simulink model "testHierCtrl"  (R2020a)
settings: Solver=ode23s  StartTime=0.0  StopTime=25  RelTol=1e-3
undefined symbols (not defined in the file or in its folder): a, courseFollowManta, courseFollowManta_cl, env, FLIGHTCONTROLLER, fltCtrl, hiLvlCtrl, initializeBussesFromBlock, vhcl
libraries: simulink x6, angleBtw2Vecs_ul x4, pathGeometry_ul x3, tanFrameProjection_ul x2, vectorNormalizer_ul x2, filteredPIDController_ul x2, velocityAngle_ul x2, eeGeneralControl x1, stopwatch_ul x1, ctrlAllocMatrix_cl x1, eulAng2RotMat_ul x1, vrlib x1
settings Model: Creator=andre  LastModifiedBy=andre
settings DataIOCC: SaveFormat=Structure

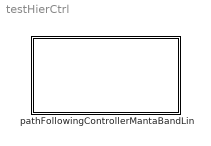
== system testHierCtrl ==
  pathFollowingControllerMantaBandLin : Subsystem  LoadFcn=initializeBussesFromBlock(gcb)  InitFcn=initializeBussesFromBlock(gcb)  StartFcn=initializeBussesFromBlock(gcb)  VariantControl=strcmpi(FLIGHTCONTROLLER,'pathFollowingControllerMantaBandLin')  mask{initPosForInitSStar=vhcl.initPosVecGnd.Value, fluidDensity=env.water.density.Value, pathCtrl=fltCtrl, aeroStruct=vhcl.struct('OCT.aeroSurf')}
      mask prompts: initPosForInitSStar "Initial Position"; fluidDensity "Fluid Density"; pathCtrl "Controller"; aeroStruct "Aerodynamic Structure"
      settings: MinAlgLoopOccurrences=on
      mask DialogControl Container3 Prompt: courseFollow Params
      mask DialogControl Container4 Prompt: setpointToOutput Params

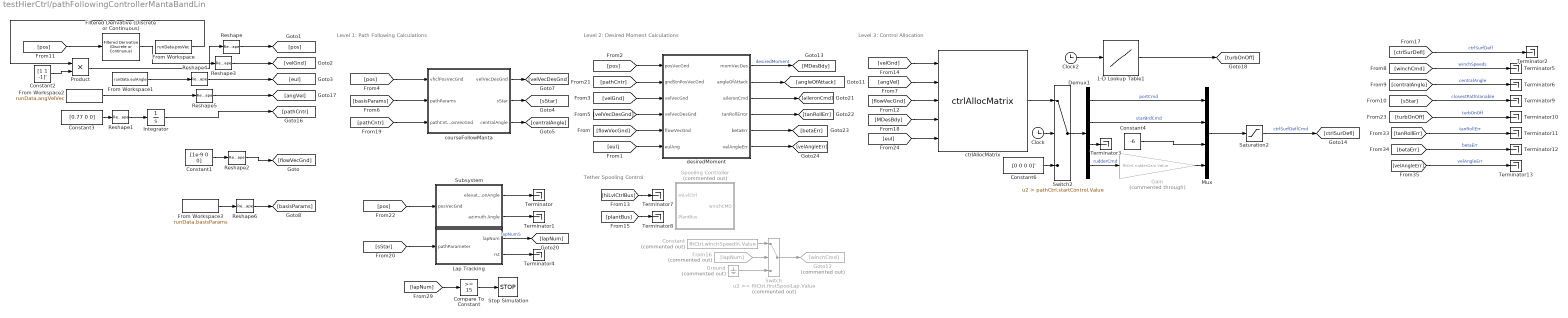
== system testHierCtrl/pathFollowingControllerMantaBandLin ==
  note: Level 1: Path Following Calculations
  note: Level 2: Desired Moment Calculations
  note: Tether Spooling Control
  note: Level 3: Control Allocation
  1-D Lookup Table1 : Lookup_n-D  NumberOfTableDimensions=1  BreakpointsForDimension1=[0 1000 2000]  Table=[0 0 0]  InterpMethod=Flat  InternalRulePriority=Speed  RndMeth=Simplest  InputSameDT=on
  Clock : Clock
  Clock2 : Clock
  Compare To Constant : simulink/Logic and Bit Operations/Compare To Constant  relop=>=  const=15  OutDataTypeStr=boolean
  Constant : Constant  Commented=on  Value=fltCtrl.winchSpeedIn.Value
  Constant1 : Constant  Value=[1e-9 0 0]
  Constant2 : Constant  Value=[1 1 -1]'
  Constant3 : Constant  Value=[0.77 0 0]
  Constant4 : Constant  Value=-6
  Constant6 : Constant  Value=[0 0 0 0]'
  Demux1 : Demux
  Filtered Derivative (Discrete or Continuous) : eeGeneralControl/Filtered Derivative (Discrete or Continuous)  K=1  T=0.1  B=inf  A=-inf  minRatio=10  init_option=Inherited from block input  x0=0  Ts=-1
      settings: SourceProductBaseCode=PS
  From Workspace : FromWorkspace  VariableName=runData.posVec
  From Workspace1 : FromWorkspace  VariableName=runData.eulAngle
  From Workspace2 : FromWorkspace  VariableName=runData.angVelVec
  From Workspace3 : FromWorkspace  VariableName=runData.basisParams
  From16 : From  Commented=on  GotoTag=lapNum
  Gain : Gain  Commented=through  Gain=fltCtrl.rudderGain.Value
  Goto12 : Goto  Commented=on  GotoTag=winchCmd
  Ground : Ground  Commented=on
  Integrator : Integrator  InitialCondition=[0 0 0]'
  Lap Tracking : Subsystem
  Mux : Mux
  Product : Product
  Reshape{,1..6} (7 alike) : Reshape  OutputDimensionality=Column vector (2-D)
  Saturation2 : Saturate  UpperLimit=pathCtrl.controlSigMax.upperLimit.Value  LowerLimit=pathCtrl.controlSigMax.lowerLimit.Value
  "Spooling Controller " : Subsystem  Commented=on
  Stop Simulation : Stop
  Subsystem : Subsystem
  Switch : Switch  Commented=on  Threshold=fltCtrl.firstSpoolLap.Value
  Switch2 : Switch  Criteria=u2 > Threshold  Threshold=pathCtrl.startControl.Value
  Terminator{,1..13} (14 alike) : Terminator
  courseFollowManta : Subsystem  AncestorBlock=courseFollowManta_cl/courseFollowManta
  ctrlAllocMatrix : ctrlAllocMatrix_cl/ctrlAllocMatrix  aeroStruct=aeroStruct  fluidDensity=fluidDensity
  desiredMoment : Subsystem
  wires:
  [velAngleErr] -> Terminator13/1  "velAngleErr"
  desiredMoment/6(velAngleErr) -> [velAngleErr]
  [betaErr] -> Terminator12/1  "betaErr"
  [tanRollErr] -> Terminator11/1  "tanRollErr"
  desiredMoment/5(betaErr) -> [betaErr]
  desiredMoment/4(tanRollError) -> [tanRollErr]
  Mux/1 -> Saturation2/1
  desiredMoment/3(aileronCmd) -> [aileronCmd]
  Compare To Constant/1 -> Stop Simulation/1
  [lapNum] -> Compare To Constant/1
  Ground/1 -> Switch/3
  Constant/1 -> Switch/1
  From16/1 -> Switch/2
  Switch/1 -> Goto12/1
  [plantBus] -> Terminator8/1
  [hiLvlCtrlBus] -> Terminator7/1
  Lap Tracking/1(lapNum) -> [lapNum]  "lapNumS"
  Lap Tracking/2(rst) -> Terminator4/1
  [sStar] -> Lap Tracking/1(pathParameter)
  Clock2/1 -> 1-D Lookup Table1/1
  1-D Lookup Table1/1 -> [turbOnOff]
  desiredMoment/2(angleOfAttack) -> [angleOfAttack]
  Constant4/1 -> Mux/3
  Subsystem/2(azimuth Angle) -> Terminator1/1
  Subsystem/1(elevationAngle) -> Terminator/1
  [pos] -> Subsystem/1(posVecGnd)
  [turbOnOff] -> Terminator10/1  "turbOnOff"
  Demux1/4 -> Gain/1  "rudderCmd"
  Gain/1 -> Mux/4
  [basisParams] -> courseFollowManta/2(pathParams)
  [flowVecGnd] -> desiredMoment/5(flowVecGnd)
  [eul] -> desiredMoment/6(eulAng)
  [velVecDesGnd] -> desiredMoment/4(velVecDesGnd)
  [velGnd] -> desiredMoment/3(velVecGnd)
  [pathCntr] -> desiredMoment/2(gndStnPosVecGnd)
  [pos] -> desiredMoment/1(posVecGnd)
  [pathCntr] -> courseFollowManta/3(pathCntrPosVecGnd)
  [eul] -> ctrlAllocMatrix/5
  Saturation2/1 -> [ctrlSurDefl]  "ctrlSurfDeflCmd"
  [ctrlSurDefl] -> Terminator2/1  "ctrlSurfDefl"
  ctrlAllocMatrix/1 -> Switch2/1
  [MDesBdy] -> ctrlAllocMatrix/4
  Constant6/1 -> Switch2/3
  Switch2/1 -> Demux1/1
  Clock/1 -> Switch2/2
  Demux1/2 -> Mux/2  "starBrdCmd"
  Demux1/1 -> Mux/1  "portCmd"
  Demux1/3 -> Terminator3/1
  [flowVecGnd] -> ctrlAllocMatrix/3
  [velGnd] -> ctrlAllocMatrix/1
  [angVel] -> ctrlAllocMatrix/2
  desiredMoment/1(momVecDes) -> [MDesBdy]  "desiredMoment"
  courseFollowManta/3(centralAngle) -> [centralAngle]
  [sStar] -> Terminator9/1  "closestPathVariable"
  [centralAngle] -> Terminator6/1  "centralAngle"
  courseFollowManta/2(sStar) -> [sStar]
  [winchCmd] -> Terminator5/1  "winchSpeeds"
  [pos] -> courseFollowManta/1("vhclPosVecGnd ")
  courseFollowManta/1(velVecDesGnd) -> [velVecDesGnd]
  From Workspace/1 -> Product/1
  Reshape3/1 -> [velGnd]
  Filtered Derivative (Discrete or Continuous)/1 -> Reshape3/1
  From Workspace1/1 -> Reshape4/1
  Constant3/1 -> Reshape1/1
  Reshape1/1 -> Integrator/1
  Integrator/1 -> [pathCntr]
  Constant1/1 -> Reshape2/1
  Reshape2/1 -> [flowVecGnd]
  Reshape/1 -> [pos]
  [pos] -> Filtered Derivative (Discrete or Continuous)/1
  From Workspace2/1 -> Reshape5/1
  From Workspace3/1 -> Reshape6/1
  Reshape4/1 -> [eul]
  Reshape5/1 -> [angVel]
  Reshape6/1 -> [basisParams]
  Constant2/1 -> Product/2
  Product/1 -> Reshape/1

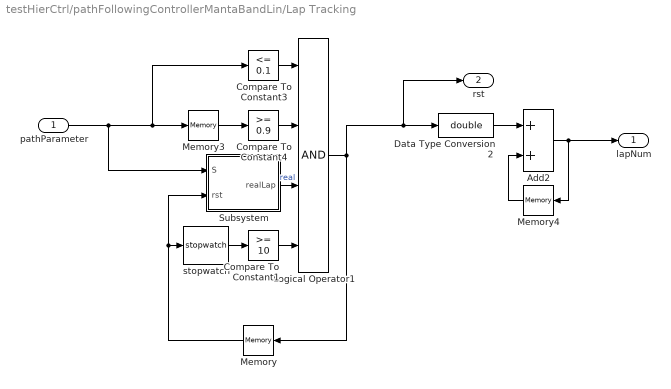
== system testHierCtrl/pathFollowingControllerMantaBandLin/Lap Tracking ==
  pathParameter : Inport
  Add2 : Sum
  Compare To Constant1 : simulink/Logic and Bit Operations/Compare To Constant  relop=>=  const=10  OutDataTypeStr=boolean
  Compare To Constant3 : simulink/Logic and Bit Operations/Compare To Constant  relop=<=  const=0.1  OutDataTypeStr=boolean
  Compare To Constant4 : simulink/Logic and Bit Operations/Compare To Constant  relop=>=  const=0.9  OutDataTypeStr=boolean
  Data Type Conversion2 : DataTypeConversion  OutDataTypeStr=double
  Logical Operator1 : Logic  Inputs=4  AllPortsSameDT=off  OutDataTypeStr=boolean
  Memory : Memory  InitialCondition=false
  Memory3 : Memory
  Memory4 : Memory
  Subsystem : Subsystem
  stopwatch : stopwatch_ul/stopwatch  SystemSampleTime=-1  Latency=0  AutoFrameSizeCalculation=off
  lapNum : Outport  VectorParamsAs1DForOutWhenUnconnected=off
  rst : Outport  Port=2  VectorParamsAs1DForOutWhenUnconnected=off
  wires:
  Subsystem/1(realLap) -> Logical Operator1/3  "real"
  Compare To Constant1/1 -> Logical Operator1/4
  Memory/1 -> stopwatch/1, Subsystem/2(rst)
  stopwatch/1 -> Compare To Constant1/1
  pathParameter/1 -> Memory3/1, Compare To Constant3/1, Subsystem/1(S)
  Compare To Constant4/1 -> Logical Operator1/2
  Add2/1 -> Memory4/1, lapNum/1
  Memory4/1 -> Add2/2
  Logical Operator1/1 -> Memory/1, Data Type Conversion2/1, rst/1
  Data Type Conversion2/1 -> Add2/1
  Memory3/1 -> Compare To Constant4/1
  Compare To Constant3/1 -> Logical Operator1/1

== system testHierCtrl/pathFollowingControllerMantaBandLin/Spooling Controller  ==
  HiLvlCtrl : Inport
  PlantBus : Inport  Port=2
  Add1 : Sum  Inputs=+-
  Bus Selector1 : BusSelector  OutputSignals=avgTetherLength
  Bus Selector3 : BusSelector  OutputSignals=basisParams
  Constant2 : Constant  Value=fltCtrl.optAltitude.Value
  Constant3 : Constant  Value=hiLvlCtrl.ThrCtrl.Value
  Fcn : Fcn  Expr=u(2)/sin(u(1))
  Ground : Ground
  Multiport Switch : MultiPortSwitch  DataPortOrder=Specify indices  Inputs=2  DataPortIndices={0,1}
  Mux1 : Mux  Inputs=2
  Saturation : Saturate  UpperLimit=.25  LowerLimit=-.25
  Selector2 : Selector  InputPortWidth=5  IndexOptions=Index vector (dialog)  Indices=3  OutputSizes=1
  winchCMD : Outport
  wires:
  PlantBus/1 -> Bus Selector1/1
  Constant3/1 -> Multiport Switch/1
  Saturation/1 -> Multiport Switch/2
  Ground/1 -> Multiport Switch/3
  HiLvlCtrl/1 -> Bus Selector3/1
  Multiport Switch/1 -> winchCMD/1  "winchCMD"
  Selector2/1 -> Mux1/1
  Fcn/1 -> Add1/1  "thrDes"
  Add1/1 -> Saturation/1
  Constant2/1 -> Mux1/2
  Bus Selector1/1 -> Add1/2  "<avgTetherLength>"
  Mux1/1 -> Fcn/1
  Bus Selector3/1 -> Selector2/1  "<basisParams>"

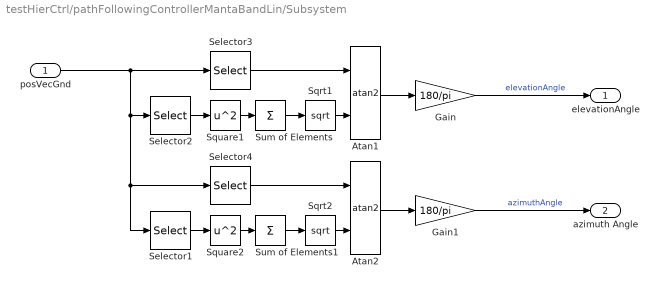
== system testHierCtrl/pathFollowingControllerMantaBandLin/Subsystem ==
  posVecGnd : Inport
  Atan1 : Trigonometry  Operator=atan2
  Atan2 : Trigonometry  Operator=atan2
  Gain : Gain  Gain=180/pi
  Gain1 : Gain  Gain=180/pi
  Selector1 : Selector  InputPortWidth=3  IndexOptions=Index vector (dialog)  Indices=1  OutputSizes=1
  Selector2 : Selector  InputPortWidth=3  IndexOptions=Index vector (dialog)  Indices=[1 2]  OutputSizes=1
  Selector3 : Selector  InputPortWidth=3  IndexOptions=Index vector (dialog)  Indices=3  OutputSizes=1
  Selector4 : Selector  InputPortWidth=3  IndexOptions=Index vector (dialog)  Indices=2  OutputSizes=1
  Sqrt1 : Sqrt  SaturateOnIntegerOverflow=on
  Sqrt2 : Sqrt  SaturateOnIntegerOverflow=on
  Square1 : Math  Operator=square  SignedPower=on  SaturateOnIntegerOverflow=on
  Square2 : Math  Operator=square  SignedPower=on  SaturateOnIntegerOverflow=on
  Sum of Elements : Sum  Inputs=+
  Sum of Elements1 : Sum  Inputs=+
  elevationAngle : Outport
  azimuth Angle : Outport  Port=2
  wires:
  Gain1/1 -> azimuth Angle/1  "azimuthAngle"
  Selector4/1 -> Atan2/1
  Sqrt2/1 -> Atan2/2
  posVecGnd/1 -> Selector3/1, Selector2/1, Selector4/1, Selector1/1
  Selector1/1 -> Square2/1
  Sum of Elements1/1 -> Sqrt2/1
  Square2/1 -> Sum of Elements1/1
  Atan2/1 -> Gain1/1
  Gain/1 -> elevationAngle/1  "elevationAngle"
  Selector2/1 -> Square1/1
  Atan1/1 -> Gain/1
  Sum of Elements/1 -> Sqrt1/1
  Selector3/1 -> Atan1/1
  Square1/1 -> Sum of Elements/1
  Sqrt1/1 -> Atan1/2

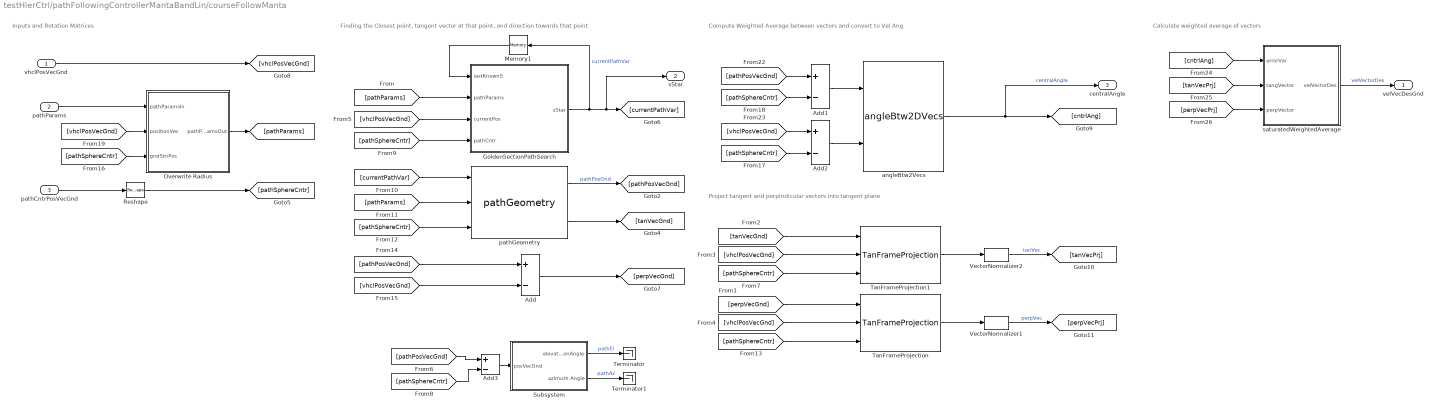
== system testHierCtrl/pathFollowingControllerMantaBandLin/courseFollowManta ==
  note: Finding the Closest point, tangent vector at that point, and direction towards that point
  note: Inputs and Rotation Matrices
  note: Compute Weighted Average between vectors and convert to Vel Ang
  note: Project tangent and perpindicular vectors into tangent plane
  note: Calculate weighted average of vectors
  "vhclPosVecGnd " : Inport
  pathParams : Inport  Port=2
  pathCntrPosVecGnd : Inport  Port=3
  Add{,1..3} (4 alike) : Sum  Inputs=+-
  GoldenSectionPathSearch : Subsystem  TreatAsAtomicUnit=on
  Memory1 : Memory
  Overwrite Radius : Subsystem
  Reshape : Reshape  OutputDimensionality=Column vector (2-D)
  Subsystem : Subsystem
  TanFrameProjection : tanFrameProjection_ul/TanFrameProjection  SystemSampleTime=-1  Latency=0  AutoFrameSizeCalculation=off
  TanFrameProjection1 : tanFrameProjection_ul/TanFrameProjection  SystemSampleTime=-1  Latency=0  AutoFrameSizeCalculation=off
  Terminator : Terminator
  Terminator1 : Terminator
  VectorNormalizer1 : vectorNormalizer_ul/VectorNormalizer   SystemSampleTime=-1  Latency=0  AutoFrameSizeCalculation=off
  VectorNormalizer2 : vectorNormalizer_ul/VectorNormalizer   SystemSampleTime=-1  Latency=0  AutoFrameSizeCalculation=off
  angleBtw2Vecs : angleBtw2Vecs_ul/angleBtw2DVecs  SystemSampleTime=-1  Latency=0  AutoFrameSizeCalculation=off
  pathGeometry : pathGeometry_ul/pathGeometry  SystemSampleTime=-1  Latency=0  AutoFrameSizeCalculation=off
  saturatedWeightedAverage : Subsystem  mask{error_upper_lim=pathCtrl.perpErrorVal.Value}
      mask prompts: error_upper_lim "Value of Error yielding 100% perpendicular"
  velVecDesGnd : Outport  VectorParamsAs1DForOutWhenUnconnected=off
  sStar : Outport  Port=2  VectorParamsAs1DForOutWhenUnconnected=off
  centralAngle : Outport  Port=3  VectorParamsAs1DForOutWhenUnconnected=off
  wires:
  saturatedWeightedAverage/1("velVectorDes ") -> velVecDesGnd/1  "velVectorDes"
  [perpVecPrj] -> saturatedWeightedAverage/3("perpVector ")
  [tanVecPrj] -> saturatedWeightedAverage/2(tangVector)
  [cntrlAng] -> saturatedWeightedAverage/1("errorVar ")
  [pathSphereCntr] -> TanFrameProjection/3
  [pathSphereCntr] -> TanFrameProjection1/3
  [vhclPosVecGnd] -> TanFrameProjection/2
  [vhclPosVecGnd] -> TanFrameProjection1/2
  [tanVecGnd] -> TanFrameProjection1/1
  [perpVecGnd] -> TanFrameProjection/1
  [vhclPosVecGnd] -> Overwrite Radius/2(positionVec)
  [pathSphereCntr] -> Overwrite Radius/3(gndStnPos)
  Add2/1 -> angleBtw2Vecs/2
  Add1/1 -> angleBtw2Vecs/1
  [pathSphereCntr] -> Add1/2
  [pathSphereCntr] -> Add2/2
  [pathSphereCntr] -> GoldenSectionPathSearch/4(pathCntr)
  [pathSphereCntr] -> pathGeometry/3
  Reshape/1 -> [pathSphereCntr]
  pathCntrPosVecGnd/1 -> Reshape/1
  Overwrite Radius/1(pathParamsOut) -> [pathParams]
  pathParams/1 -> Overwrite Radius/1(pathParamsIn)
  TanFrameProjection/1 -> VectorNormalizer1/1
  pathGeometry/2 -> [tanVecGnd]
  [pathPosVecGnd] -> Add/1
  [vhclPosVecGnd] -> Add/2
  Add/1 -> [perpVecGnd]
  Memory1/1 -> GoldenSectionPathSearch/1(lastKnownS)
  GoldenSectionPathSearch/1(sStar) -> [currentPathVar], sStar/1, Memory1/1  "currentPathVar"
  [pathParams] -> GoldenSectionPathSearch/2(pathParams)
  TanFrameProjection1/1 -> VectorNormalizer2/1
  [currentPathVar] -> pathGeometry/1
  [vhclPosVecGnd] -> Add2/1
  angleBtw2Vecs/1 -> centralAngle/1, [cntrlAng]  "centralAngle"
  VectorNormalizer1/1 -> [perpVecPrj]  "perpVec"
  [pathParams] -> pathGeometry/2
  pathGeometry/1 -> [pathPosVecGnd]  "pathPosGnd"
  "vhclPosVecGnd "/1 -> [vhclPosVecGnd]
  [vhclPosVecGnd] -> GoldenSectionPathSearch/3(currentPos)
  VectorNormalizer2/1 -> [tanVecPrj]  "tanVec"
  [pathPosVecGnd] -> Add1/1
  [pathPosVecGnd] -> Add3/1
  Subsystem/1(elevationAngle) -> Terminator/1  "pathEl"
  Subsystem/2(azimuth Angle) -> Terminator1/1  "pathAz"
  Add3/1 -> Subsystem/1(posVecGnd)
  [pathSphereCntr] -> Add3/2

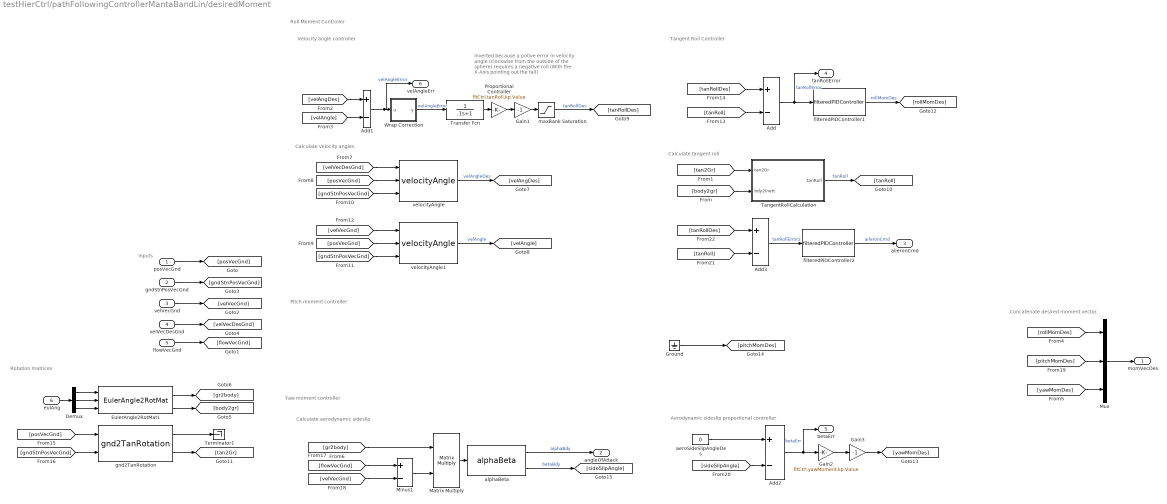
== system testHierCtrl/pathFollowingControllerMantaBandLin/desiredMoment ==
  note: Calculate aerodynamic sideslip
  note: Aerodynamic sideslip proportional controller
  note: Roll Moment Controller
  note: Concatenate desired moment vector
  note: Tangent Roll Controller
  note: Calculate tangent roll
  note: Calculate velocity angles
  note: Rotation matrices
  note: Inputs
  note: Velocity angle controller
  note: Inverted because a potive error
      | in velocity angle (clockwise from the
      | outside of the sphere) requires a negative
      | roll (With the X-Axis pointing out the tail)
  note: Pitch moment controller
  note: Yaw moment controller
  posVecGnd : Inport
  gndStnPosVecGnd : Inport  Port=2
  velVecGnd : Inport  Port=3
  velVecDesGnd : Inport  Port=4
  flowVecGnd : Inport  Port=5
  eulAng : Inport  Port=6
  Add{,1..3} (4 alike) : Sum  Inputs=+-
  Demux : Demux  Outputs=3
  EulerAngle2RotMat1 : eulAng2RotMat_ul/EulerAngle2RotMat  SystemSampleTime=-1  Latency=0  AutoFrameSizeCalculation=off
  Gain1 : Gain  Gain=-1
  Gain2 : Gain  Gain=fltCtrl.yawMoment.kp.Value
  Gain3 : Gain  Gain=-1
  Ground : Ground
  Matrix Multiply : Product  Multiplication=Matrix(*)
  Minus1 : Sum  Inputs=+-
  Mux : Mux  Inputs=3
  Proportional Controller : Gain  Gain=fltCtrl.tanRoll.kp.Value
  TangentRollCalculation : Subsystem
  Terminator1 : Terminator
  Transfer Fcn : TransferFcn  Denominator=[.1 1]
  Wrap Correction : Subsystem
  aeroSideSlipAngleDes : Constant  Value=0
  alphaBeta : alphaBeta_ul/alphaBeta  SystemSampleTime=-1  Latency=0  AutoFrameSizeCalculation=off
  filteredPIDController1 : filteredPIDController_ul/filteredPIDController  kp=pathCtrl.rollMoment.kp.Value  ki=0  kd=pathCtrl.rollMoment.kd.Value  Value=pathCtrl.rollMoment.tau.Value  externalReset=none
  filteredPIDController2 : filteredPIDController_ul/filteredPIDController  kp=fltCtrl.rollCtrl.kp.Value  ki=fltCtrl.rollCtrl.ki.Value  kd=fltCtrl.rollCtrl.kd.Value  Value=fltCtrl.rollCtrl.tau.Value  externalReset=none
  gnd2TanRotation : gnd2TanRotation_ul/gnd2TanRotation  SystemSampleTime=-1  Latency=0  AutoFrameSizeCalculation=off
  maxBank Saturation : Saturate  UpperLimit=pathCtrl.maxBank.upperLimit.Value  LowerLimit=pathCtrl.maxBank.lowerLimit.Value
  velocityAngle : velocityAngle_ul/velocityAngle  SystemSampleTime=-1  Latency=0  AutoFrameSizeCalculation=off
  velocityAngle1 : velocityAngle_ul/velocityAngle  SystemSampleTime=-1  Latency=0  AutoFrameSizeCalculation=off
  momVecDes : Outport  VectorParamsAs1DForOutWhenUnconnected=off
  angleOfAttack : Outport  Port=2  VectorParamsAs1DForOutWhenUnconnected=off
  aileronCmd : Outport  Port=3  VectorParamsAs1DForOutWhenUnconnected=off
  tanRollError : Outport  Port=4
  betaErr : Outport  Port=5
  velAngleErr : Outport  Port=6
  wires:
  filteredPIDController2/1 -> aileronCmd/1  "aileronCmd"
  [tanRollDes] -> Add3/1
  [tanRoll] -> Add3/2
  Add3/1 -> filteredPIDController2/1  "tanRollError2"
  Transfer Fcn/1 -> Proportional Controller/1
  Wrap Correction/1(y) -> Transfer Fcn/1  "velAngleError"
  Ground/1 -> [pitchMomDes]
  posVecGnd/1 -> [posVecGnd]
  velVecGnd/1 -> [velVecGnd]
  Add/1 -> filteredPIDController1/1, tanRollError/1  "tanRollError"
  Proportional Controller/1 -> Gain1/1
  Gain1/1 -> maxBank Saturation/1
  maxBank Saturation/1 -> [tanRollDes]  "tanRollDes"
  Add1/1 -> velAngleErr/1, Wrap Correction/1(u)  "velAngleError"
  flowVecGnd/1 -> [flowVecGnd]
  [tan2Gr] -> TangentRollCalculation/1(tan2Gr)
  TangentRollCalculation/1(tanRoll) -> [tanRoll]  "tanRoll"
  filteredPIDController1/1 -> [rollMomDes]  "rollMomDes"
  Gain2/1 -> Gain3/1
  Minus1/1 -> Matrix Multiply/2
  [velVecGnd] -> Minus1/2
  [flowVecGnd] -> Minus1/1
  eulAng/1 -> Demux/1
  Demux/3 -> EulerAngle2RotMat1/3
  Demux/1 -> EulerAngle2RotMat1/1
  Demux/2 -> EulerAngle2RotMat1/2
  EulerAngle2RotMat1/2 -> [body2gr]
  EulerAngle2RotMat1/1 -> [gr2body]
  [body2gr] -> TangentRollCalculation/2(bdy2Inert)
  [gr2body] -> Matrix Multiply/1
  Matrix Multiply/1 -> alphaBeta/1
  alphaBeta/2 -> [sideSlipAngle]  "betaBdy"
  Add2/1 -> Gain2/1, betaErr/1  "betaErr"
  aeroSideSlipAngleDes/1 -> Add2/1
  Mux/1 -> momVecDes/1
  Gain3/1 -> [yawMomDes]
  alphaBeta/1 -> angleOfAttack/1  "alphaBdy"
  [pitchMomDes] -> Mux/2
  gndStnPosVecGnd/1 -> [gndStnPosVecGnd]
  velVecDesGnd/1 -> [velVecDesGnd]
  velocityAngle/1 -> [velAngDes]  "velAngleDes"
  velocityAngle1/1 -> [velAngle]  "velAngle"
  [velAngDes] -> Add1/1
  [velAngle] -> Add1/2
  [velVecDesGnd] -> velocityAngle/1
  [posVecGnd] -> velocityAngle/2
  [posVecGnd] -> velocityAngle1/2
  [gndStnPosVecGnd] -> velocityAngle/3
  [gndStnPosVecGnd] -> velocityAngle1/3
  [velVecGnd] -> velocityAngle1/1
  [tanRoll] -> Add/2
  [tanRollDes] -> Add/1
  [posVecGnd] -> gnd2TanRotation/1
  [gndStnPosVecGnd] -> gnd2TanRotation/2
  gnd2TanRotation/2 -> [tan2Gr]
  gnd2TanRotation/1 -> Terminator1/1
  [rollMomDes] -> Mux/1
  [yawMomDes] -> Mux/3
  [sideSlipAngle] -> Add2/2

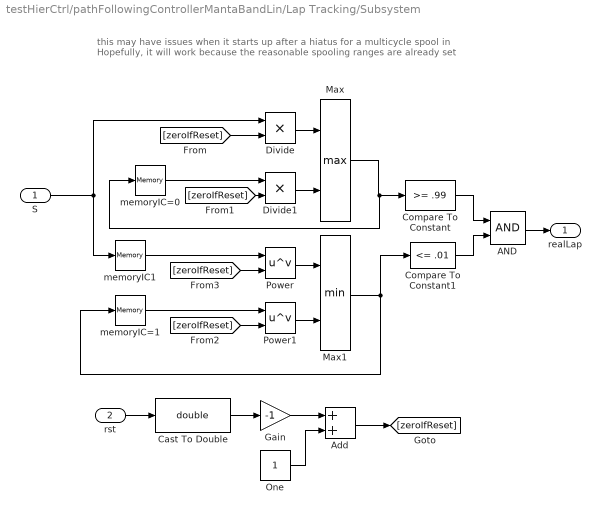
== system testHierCtrl/pathFollowingControllerMantaBandLin/Lap Tracking/Subsystem ==
  note: this may have issues when it starts up after a hiatus for a multicycle spool in
      | Hopefully, it will work because the reasonable spooling ranges are already set
  S : Inport
  rst : Inport  Port=2
  AND : Logic  AllPortsSameDT=off  OutDataTypeStr=boolean
  Add : Sum
  Cast To Double : DataTypeConversion  OutDataTypeStr=double
  Compare To Constant : simulink/Logic and Bit Operations/Compare To Constant  relop=>=  const=.99  OutDataTypeStr=boolean
  Compare To Constant1 : simulink/Logic and Bit Operations/Compare To Constant  relop=<=  const=.01  OutDataTypeStr=boolean
  Divide : Product  Inputs=**
  Divide1 : Product  Inputs=**
  Gain : Gain  Gain=-1
  Max : MinMax  Function=max  Inputs=2
  Max1 : MinMax  Inputs=2
  One : Constant  OutDataTypeStr=Inherit: Inherit via back propagation
  Power : Math  Operator=pow  SaturateOnIntegerOverflow=on
  Power1 : Math  Operator=pow  SaturateOnIntegerOverflow=on
  memoryIC1 : Memory  InitialCondition=1
  memoryIC=0 : Memory
  memoryIC=1 : Memory  InitialCondition=1
  realLap : Outport
  wires:
  memoryIC1/1 -> Power/1
  memoryIC=1/1 -> Power1/1
  [zeroIfReset] -> Power1/2
  memoryIC=0/1 -> Divide1/1
  Divide1/1 -> Max/2
  [zeroIfReset] -> Divide1/2
  [zeroIfReset] -> Power/2
  [zeroIfReset] -> Divide/2
  AND/1 -> realLap/1
  Compare To Constant1/1 -> AND/2
  Compare To Constant/1 -> AND/1
  Cast To Double/1 -> Gain/1
  Power1/1 -> Max1/2
  Power/1 -> Max1/1
  Max/1 -> Compare To Constant/1, memoryIC=0/1
  Divide/1 -> Max/1
  One/1 -> Add/2
  Add/1 -> [zeroIfReset]
  Gain/1 -> Add/1
  S/1 -> memoryIC1/1, Divide/1
  rst/1 -> Cast To Double/1
  Max1/1 -> memoryIC=1/1, Compare To Constant1/1

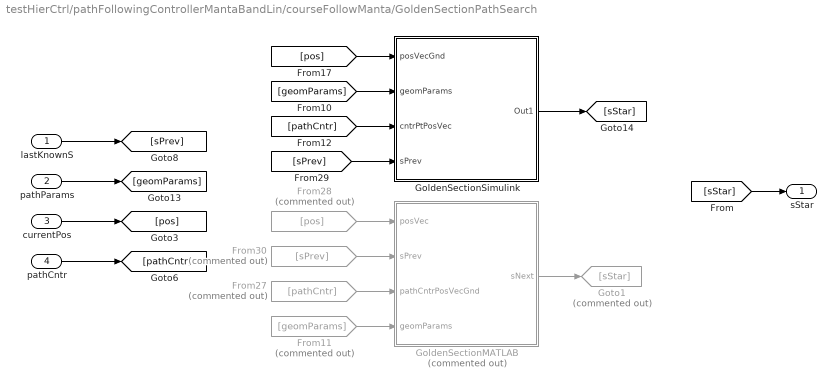
== system testHierCtrl/pathFollowingControllerMantaBandLin/courseFollowManta/GoldenSectionPathSearch ==
  lastKnownS : Inport
  pathParams : Inport  Port=2
  currentPos : Inport  Port=3
  pathCntr : Inport  Port=4
  From11 : From  Commented=on  GotoTag=geomParams
  From27 : From  Commented=on  GotoTag=pathCntr
  From28 : From  Commented=on  GotoTag=pos
  From30 : From  Commented=on  GotoTag=sPrev
  GoldenSectionMATLAB : MATLAB Function  Commented=on  TreatAsAtomicUnit=on  mask{geomFunc=pathCtrl, searchWidth=0.1, pathVarTol=1e-5}
  GoldenSectionSimulink : Subsystem
  Goto1 : Goto  Commented=on  GotoTag=sStar
  sStar : Outport  InitialOutput=pathCtrl.initPathVar.Value  VectorParamsAs1DForOutWhenUnconnected=off
  wires:
  GoldenSectionSimulink/1(Out1) -> [sStar]
  [sPrev] -> GoldenSectionSimulink/4(sPrev)
  [pathCntr] -> GoldenSectionSimulink/3(cntrPtPosVec)
  [geomParams] -> GoldenSectionSimulink/2(geomParams)
  [pos] -> GoldenSectionSimulink/1(posVecGnd)
  [sStar] -> sStar/1
  lastKnownS/1 -> [sPrev]
  From27/1 -> GoldenSectionMATLAB/3(pathCntrPosVecGnd)
  From30/1 -> GoldenSectionMATLAB/2(sPrev)
  From28/1 -> GoldenSectionMATLAB/1(posVec)
  From11/1 -> GoldenSectionMATLAB/4(geomParams)
  GoldenSectionMATLAB/1(sNext) -> Goto1/1
  pathCntr/1 -> [pathCntr]
  pathParams/1 -> [geomParams]
  currentPos/1 -> [pos]

== system testHierCtrl/pathFollowingControllerMantaBandLin/courseFollowManta/Overwrite Radius ==
  note: subsystem overwrites the 5th basis parameter with the current radius
      | so that the downstream blocks calculate the path geomatry at the current radius.
  pathParamsIn : Inport
  positionVec : Inport  Port=2
  gndStnPos : Inport  Port=3
  Add : Sum  Inputs=+-
  Assignment : Assignment  NumberOfDimensions=2  DiagnosticForDimensions=Warning  IndexOptions=Index vector (dialog),Assign all  Indices=5,5  OutputSizes=1,1
  Dot Product : DotProduct  InputSameDT=on  OutDataTypeStr=Inherit: Inherit via internal rule
  Sqrt : Sqrt  SaturateOnIntegerOverflow=on
  pathParamsOut : Outport  VectorParamsAs1DForOutWhenUnconnected=off
  wires:
  gndStnPos/1 -> Add/2
  positionVec/1 -> Add/1
  pathParamsIn/1 -> Assignment/1
  Sqrt/1 -> Assignment/2
  Assignment/1 -> pathParamsOut/1
  Dot Product/1 -> Sqrt/1
  Add/1 -> Dot Product/1, Dot Product/2

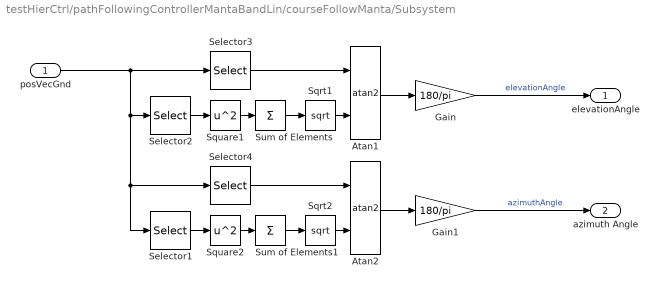
== system testHierCtrl/pathFollowingControllerMantaBandLin/courseFollowManta/Subsystem ==
  posVecGnd : Inport
  Atan1 : Trigonometry  Operator=atan2
  Atan2 : Trigonometry  Operator=atan2
  Gain : Gain  Gain=180/pi
  Gain1 : Gain  Gain=180/pi
  Selector1 : Selector  InputPortWidth=3  IndexOptions=Index vector (dialog)  Indices=1  OutputSizes=1
  Selector2 : Selector  InputPortWidth=3  IndexOptions=Index vector (dialog)  Indices=[1 2]  OutputSizes=1
  Selector3 : Selector  InputPortWidth=3  IndexOptions=Index vector (dialog)  Indices=3  OutputSizes=1
  Selector4 : Selector  InputPortWidth=3  IndexOptions=Index vector (dialog)  Indices=2  OutputSizes=1
  Sqrt1 : Sqrt  SaturateOnIntegerOverflow=on
  Sqrt2 : Sqrt  SaturateOnIntegerOverflow=on
  Square1 : Math  Operator=square  SignedPower=on  SaturateOnIntegerOverflow=on
  Square2 : Math  Operator=square  SignedPower=on  SaturateOnIntegerOverflow=on
  Sum of Elements : Sum  Inputs=+
  Sum of Elements1 : Sum  Inputs=+
  elevationAngle : Outport
  azimuth Angle : Outport  Port=2
  wires:
  Gain1/1 -> azimuth Angle/1  "azimuthAngle"
  Selector4/1 -> Atan2/1
  Sqrt2/1 -> Atan2/2
  posVecGnd/1 -> Selector3/1, Selector2/1, Selector4/1, Selector1/1
  Selector1/1 -> Square2/1
  Sum of Elements1/1 -> Sqrt2/1
  Square2/1 -> Sum of Elements1/1
  Atan2/1 -> Gain1/1
  Gain/1 -> elevationAngle/1  "elevationAngle"
  Selector2/1 -> Square1/1
  Atan1/1 -> Gain/1
  Sum of Elements/1 -> Sqrt1/1
  Selector3/1 -> Atan1/1
  Square1/1 -> Sum of Elements/1
  Sqrt1/1 -> Atan1/2

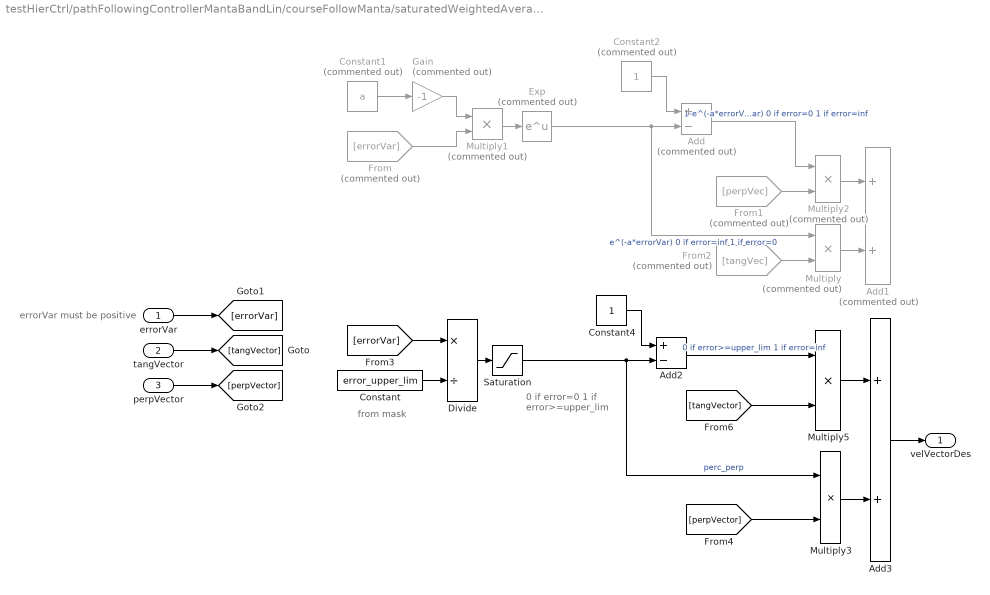
== system testHierCtrl/pathFollowingControllerMantaBandLin/courseFollowManta/saturatedWeightedAverage ==
  note: 0 if error=0
      | 1 if error>=upper_lim
  note: from mask
  note: errorVar must be positive
  "errorVar " : Inport
  tangVector : Inport  Port=2
  "perpVector " : Inport  Port=3
  Add : Sum  Commented=on  Inputs=+-
  Add1 : Sum  Commented=on
  Add2 : Sum  Inputs=+-
  Add3 : Sum
  Constant : Constant  Value=error_upper_lim
  Constant1 : Constant  Commented=on  Value=a
  Constant2 : Constant  Commented=on
  Constant4 : Constant
  Divide : Product  Inputs=*/
  Exp : Math  Commented=on  SignedPower=on  SaturateOnIntegerOverflow=on
  From : From  Commented=on  GotoTag=errorVar
  From1 : From  Commented=on  GotoTag=perpVec
  From2 : From  Commented=on  GotoTag=tangVec
  Gain : Gain  Commented=on  Gain=-1
  Multiply : Product  Commented=on
  Multiply1 : Product  Commented=on
  Multiply2 : Product  Commented=on
  Multiply3 : Product
  Multiply5 : Product
  Saturation : Saturate  UpperLimit=1  LowerLimit=0
  "velVectorDes " : Outport  VectorParamsAs1DForOutWhenUnconnected=off
  wires:
  tangVector/1 -> [tangVector]
  Constant1/1 -> Gain/1
  Gain/1 -> Multiply1/1
  Multiply1/1 -> Exp/1
  Exp/1 -> Multiply/1, Add/2  "e^(-a*errorVar) 0 if error=inf 1 if error=0"
  Constant2/1 -> Add/1
  Add/1 -> Multiply2/1  "1-e^(-a*errorVar) 0 if error=0 1 if error=inf"
  "errorVar "/1 -> [errorVar]
  "perpVector "/1 -> [perpVector]
  From/1 -> Multiply1/2
  Multiply2/1 -> Add1/1
  Multiply/1 -> Add1/2
  From1/1 -> Multiply2/2
  From2/1 -> Multiply/2
  Constant4/1 -> Add2/1
  Saturation/1 -> Multiply3/1, Add2/2  "perc_perp"
  Add3/1 -> "velVectorDes "/1
  Multiply3/1 -> Add3/2
  Multiply5/1 -> Add3/1
  Add2/1 -> Multiply5/1  "0 if error>=upper_lim 1 if error=inf"
  [errorVar] -> Divide/1
  Constant/1 -> Divide/2
  Divide/1 -> Saturation/1
  [tangVector] -> Multiply5/2
  [perpVector] -> Multiply3/2

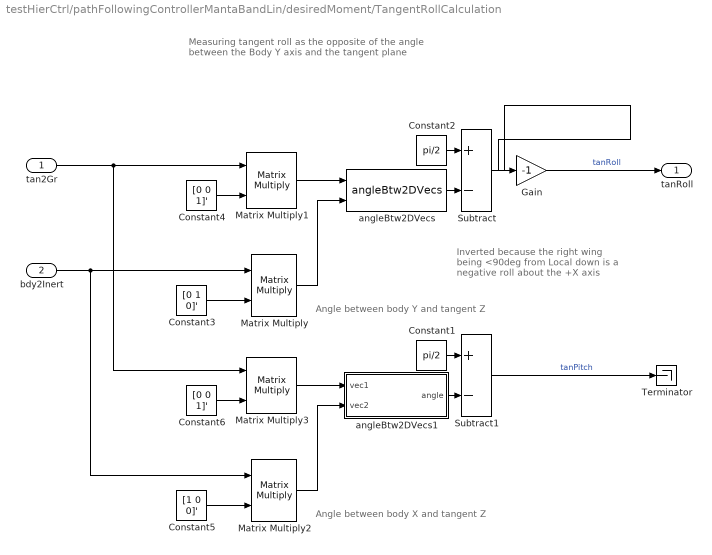
== system testHierCtrl/pathFollowingControllerMantaBandLin/desiredMoment/TangentRollCalculation ==
  note: Measuring tangent roll as the opposite
      | of the angle between the Body Y axis
      | and the tangent plane
  note: Angle between body Y and tangent Z
  note: Inverted because the right wing
      | being <90deg from Local down
      | is a negative roll about the +X axis
  note: Angle between body X and tangent Z
  tan2Gr : Inport
  bdy2Inert : Inport  Port=2
  Constant1 : Constant  Value=pi/2
  Constant2 : Constant  Value=pi/2
  Constant3 : Constant  Value=[0 1 0]'
  Constant4 : Constant  Value=[0 0 1]'
  Constant5 : Constant  Value=[1 0 0]'
  Constant6 : Constant  Value=[0 0 1]'
  Gain : Gain  Gain=-1
  Matrix Multiply{,1..3} (4 alike) : Product  Multiplication=Matrix(*)
  Subtract : Sum  Inputs=+-
  Subtract1 : Sum  Inputs=+-
  Terminator : Terminator
  angleBtw2DVecs : angleBtw2Vecs_ul/angleBtw2DVecs  SystemSampleTime=-1  Latency=0  AutoFrameSizeCalculation=off
  angleBtw2DVecs1 : Subsystem
  tanRoll : Outport  VectorParamsAs1DForOutWhenUnconnected=off
  wires:
  Subtract/1 -> Gain/1
  Constant3/1 -> Matrix Multiply/2
  angleBtw2DVecs/1 -> Subtract/2
  Constant2/1 -> Subtract/1
  Matrix Multiply1/1 -> angleBtw2DVecs/1
  Constant4/1 -> Matrix Multiply1/2
  Matrix Multiply/1 -> angleBtw2DVecs/2
  Gain/1 -> tanRoll/1  "tanRoll"
  bdy2Inert/1 -> Matrix Multiply2/1, Matrix Multiply/1
  Subtract1/1 -> Terminator/1  "tanPitch"
  tan2Gr/1 -> Matrix Multiply3/1, Matrix Multiply1/1
  Matrix Multiply2/1 -> angleBtw2DVecs1/2(vec2)
  Constant6/1 -> Matrix Multiply3/2
  Matrix Multiply3/1 -> angleBtw2DVecs1/1(vec1)
  Constant1/1 -> Subtract1/1
  angleBtw2DVecs1/1(angle) -> Subtract1/2
  Constant5/1 -> Matrix Multiply2/2

== system testHierCtrl/pathFollowingControllerMantaBandLin/desiredMoment/Wrap Correction ==
  note: output = mod(input-pi,2*pi)-pi
      | wraps output to -pi to pi
      |
      | ex) 1.5*pi will become -.5pi
      | 	and -1.5pi will become .5pi
      |
      | to visualize, plot the fuction above
  u : Inport
  Add1 : Sum  Inputs=+-
  Add2 : Sum  Inputs=+-
  Constant1 : Constant  Value=pi
  Constant2 : Constant  Value=2*pi
  Constant3 : Constant  Value=pi
  Mod : Math  Operator=mod  SignedPower=on  SaturateOnIntegerOverflow=on
  y : Outport  VectorParamsAs1DForOutWhenUnconnected=off
  wires:
  u/1 -> Add1/1
  Constant1/1 -> Add1/2
  Add1/1 -> Mod/1
  Constant2/1 -> Mod/2
  Mod/1 -> Add2/1  "always_pos"
  Constant3/1 -> Add2/2
  Add2/1 -> y/1

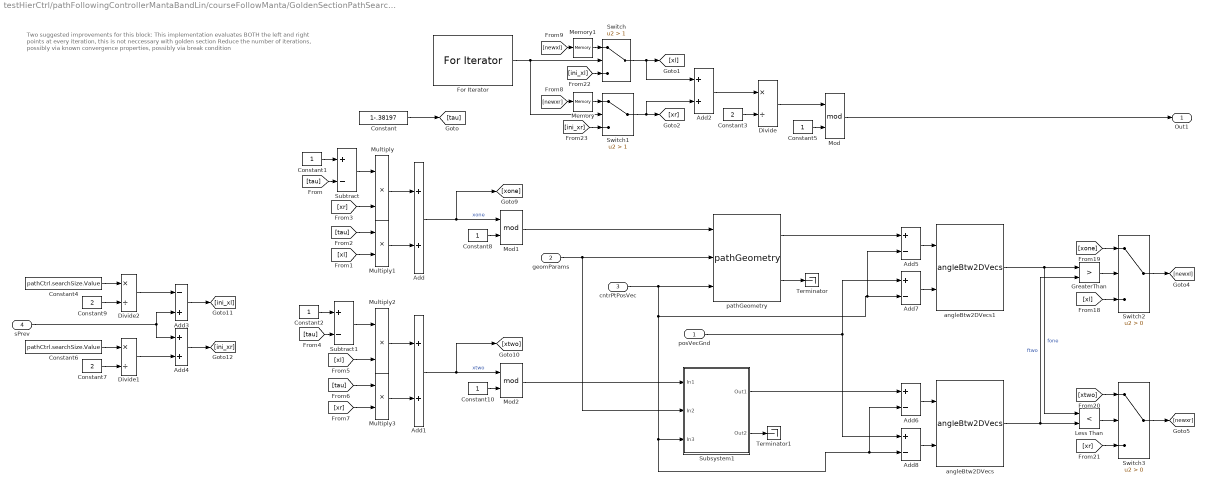
== system testHierCtrl/pathFollowingControllerMantaBandLin/courseFollowManta/GoldenSectionPathSearch/GoldenSectionSimulink ==
  note: Two suggested improvements for this block:
      | This implementation evaluates BOTH the left and right points at every iteration, this is not neccessary with golden section
      | Reduce the number of iterations, possibly via known convergence properties, possibly via break condition
  posVecGnd : Inport
  geomParams : Inport  Port=2
  cntrPtPosVec : Inport  Port=3
  sPrev : Inport  Port=4
  Add{,1..2,4} (4 alike) : Sum
  Add3 : Sum  Inputs=-+
  Add{5..8} (4 alike) : Sum  Inputs=+-
  Constant : Constant  Value=1-.38197
  Constant{1..2,5,8,10} (5 alike) : Constant
  Constant3 : Constant  Value=2
  Constant4 : Constant  Value=pathCtrl.searchSize.Value
  Constant6 : Constant  Value=pathCtrl.searchSize.Value
  Constant7 : Constant  Value=2
  Constant9 : Constant  Value=2
  Divide : Product  Inputs=*/
  Divide1 : Product  Inputs=*/
  Divide2 : Product  Inputs=*/
  For Iterator : ForIterator  IterationLimit=25
  GreaterThan : RelationalOperator  Operator=>  OutDataTypeStr=boolean  RndMeth=Simplest
  Less Than : RelationalOperator  Operator=<  OutDataTypeStr=boolean  RndMeth=Simplest
  Memory : Memory  InheritSampleTime=on
  Memory1 : Memory  InheritSampleTime=on
  Mod : Math  Operator=mod  SignedPower=on  SaturateOnIntegerOverflow=on
  Mod1 : Math  Operator=mod  SignedPower=on  SaturateOnIntegerOverflow=on
  Mod2 : Math  Operator=mod  SignedPower=on  SaturateOnIntegerOverflow=on
  Multiply{,1..3} (4 alike) : Product
  Subsystem1 : Subsystem
  Subtract : Sum  Inputs=+-
  Subtract1 : Sum  Inputs=+-
  Switch : Switch  Criteria=u2 > Threshold  Threshold=1
  Switch1 : Switch  Criteria=u2 > Threshold  Threshold=1
  Switch2 : Switch  Criteria=u2 > Threshold
  Switch3 : Switch  Criteria=u2 > Threshold
  Terminator : Terminator
  Terminator1 : Terminator
  angleBtw2DVecs : angleBtw2Vecs_ul/angleBtw2DVecs  SystemSampleTime=-1  Latency=0  AutoFrameSizeCalculation=off
  angleBtw2DVecs1 : angleBtw2Vecs_ul/angleBtw2DVecs  SystemSampleTime=-1  Latency=0  AutoFrameSizeCalculation=off
  pathGeometry : pathGeometry_ul/pathGeometry  SystemSampleTime=-1  Latency=0  AutoFrameSizeCalculation=off
  Out1 : Outport
  wires:
  Add8/1 -> angleBtw2DVecs/2
  Multiply1/1 -> Add/2
  Switch3/1 -> [newxr]
  [ini_xl] -> Switch/3
  Mod/1 -> Out1/1
  Divide2/1 -> Add3/1
  Switch2/1 -> [newxl]
  pathGeometry/2 -> Terminator/1
  [newxl] -> Memory1/1
  Constant6/1 -> Divide1/1
  Add6/1 -> angleBtw2DVecs/1
  Constant10/1 -> Mod2/2
  Add2/1 -> Divide/1
  [xl] -> Switch2/3
  [xr] -> Switch3/3
  Divide/1 -> Mod/1
  [xl] -> Multiply2/2
  Multiply3/1 -> Add1/2
  Add5/1 -> angleBtw2DVecs1/1
  sPrev/1 -> Add3/2, Add4/1
  Less Than/1 -> Switch3/2
  Constant3/1 -> Divide/2
  Add4/1 -> [ini_xr]
  Constant9/1 -> Divide2/2
  [xr] -> Multiply/2
  Add3/1 -> [ini_xl]
  Divide1/1 -> Add4/2
  Mod1/1 -> pathGeometry/1
  Memory/1 -> Switch1/1
  [newxr] -> Memory/1
  Add7/1 -> angleBtw2DVecs1/2
  [tau] -> Multiply1/1
  [xone] -> Switch2/1
  [ini_xr] -> Switch1/3
  angleBtw2DVecs1/1 -> GreaterThan/1, Less Than/1  "fone"
  Constant4/1 -> Divide2/1
  Mod2/1 -> Subsystem1/1(In1)
  Multiply2/1 -> Add1/1
  Switch1/1 -> [xr], Add2/2
  Constant/1 -> [tau]
  Add/1 -> Mod1/1, [xone]  "xone"
  For Iterator/1 -> Switch/2, Switch1/2
  Memory1/1 -> Switch/1
  [tau] -> Multiply3/1
  [tau] -> Subtract/2
  [xtwo] -> Switch3/1
  Multiply/1 -> Add/1
  [xl] -> Multiply1/2
  Subsystem1/2(Out2) -> Terminator1/1
  Subtract/1 -> Multiply/1
  Constant7/1 -> Divide1/2
  Add1/1 -> Mod2/1, [xtwo]  "xtwo"
  [tau] -> Subtract1/2
  angleBtw2DVecs/1 -> Less Than/2, GreaterThan/2  "ftwo"
  Constant5/1 -> Mod/2
  Constant1/1 -> Subtract/1
  posVecGnd/1 -> Add7/1, Add8/1
  GreaterThan/1 -> Switch2/2
  pathGeometry/1 -> Add5/1
  Constant8/1 -> Mod1/2
  [xr] -> Multiply3/2
  Subsystem1/1(Out1) -> Add6/1
  Constant2/1 -> Subtract1/1
  geomParams/1 -> Subsystem1/2(In2), pathGeometry/2
  Switch/1 -> [xl], Add2/1
  cntrPtPosVec/1 -> pathGeometry/3, Add7/2, Add5/2, Subsystem1/3(In3), Add8/2, Add6/2
  Subtract1/1 -> Multiply2/1

== system testHierCtrl/pathFollowingControllerMantaBandLin/desiredMoment/TangentRollCalculation/angleBtw2DVecs1 ==
  vec1 : Inport
  vec2 : Inport  Port=2
  Abs : Abs
  Atan2 : Trigonometry  Operator=atan2
  Cross Product : vrlib/Utilities/Cross Product
      settings: SourceProductBaseCode=VR
  Dot Product : DotProduct  InputSameDT=on  OutDataTypeStr=Inherit: Inherit via internal rule
  Dot Product1 : DotProduct  InputSameDT=on  OutDataTypeStr=Inherit: Inherit via internal rule
  Sqrt : Sqrt  SaturateOnIntegerOverflow=on
  angle : Outport  VectorParamsAs1DForOutWhenUnconnected=off
  wires:
  Atan2/1 -> Abs/1
  vec1/1 -> Dot Product/1, Cross Product/2
  vec2/1 -> Cross Product/1, Dot Product/2
  Cross Product/1 -> Dot Product1/1, Dot Product1/2
  Dot Product/1 -> Atan2/2
  Abs/1 -> angle/1
  Dot Product1/1 -> Sqrt/1
  Sqrt/1 -> Atan2/1

== system testHierCtrl/pathFollowingControllerMantaBandLin/courseFollowManta/GoldenSectionPathSearch/GoldenSectionSimulink/Subsystem1 ==
  In1 : Inport
  In2 : Inport  Port=2
  In3 : Inport  Port=3
  pathGeometry : pathGeometry_ul/pathGeometry  SystemSampleTime=-1  Latency=0  AutoFrameSizeCalculation=off
  Out1 : Outport  VectorParamsAs1DForOutWhenUnconnected=off
  Out2 : Outport  Port=2  VectorParamsAs1DForOutWhenUnconnected=off
  wires:
  pathGeometry/2 -> Out2/1
  In1/1 -> pathGeometry/1
  In3/1 -> pathGeometry/3
  pathGeometry/1 -> Out1/1
  In2/1 -> pathGeometry/2

== matlab function testHierCtrl/pathFollowingControllerMantaBandLin/courseFollowManta/GoldenSectionPathSearch/GoldenSectionMATLAB ==
  data: posVec input; sNext output; sPrev input; pathCntrPosVecGnd input; pathVarTol parameter; searchWidth parameter; geomParams input
function sNext = fcn(posVec,sPrev,pathCntrPosVecGnd, pathVarTol, searchWidth, geomParams)
% I wrote this function on 4/22/2020 when attempting to figure out some
% issues with numerical stiffness.  Turns out that althought the profiler
% was telling me the problem was with the simulink in the equivalent
% subsystem, that was a lie.  Anyways, I thought I should leave this here
% anyways just in case anyone wants to reference it.  Note that this
% implementation doesn't allow for different paths without changing
% function J below.  Which isn't great for a long term solution, so don't
% just use this as-is if you want to go to a matlab-based golden section
% implementation in the future. Also, I think there are some hard-coded
% numbers in the mask in the model, so fix that.  Finally, note that even
% though the "equivalent" simulink implementation has some inefficiencies
% that this code doesnt (as noted in the simulink implementation), there
% doesn't appear to be a siginificant difference in run times, although I
% haven't done a thorough study. -Mitchell

% phi = (sqrt(5) + 1) / 2;
% gr = 1/((1/phi)+1);
% gr = 0.618033988749895;
x1 = sPrev - searchWidth/2;
x4 = sPrev + searchWidth/2;
x2 = x4 - (x4-x1)*0.618033988749895;
x3 = x1 + (x4-x1)*0.618033988749895;
% J1 = J(x1,posVec,geomParams,pathCntrPosVecGnd);
J2 = J(x2,posVec,geomParams,pathCntrPosVecGnd);
J3 = J(x3,posVec,geomParams,pathCntrPosVecGnd);
% J4 = J(x4,posVec,geomParams,pathCntrPosVecGnd);
% JL =JFunc(xL);
% JR = JFunc(xR);
% plot([x1 x2 x3 x4],[J1 J2 J3 J4])
for ii = 1:100 
    if J2<J3
        x4 = x3;
%         J4 = J(x4,posVec,geomParams,pathCntrPosVecGnd);
        x3 = x2;
        J3 = J2;
        x2 = x4 - (x4-x1)*0.618033988749895;
        J2 = J(x2,posVec,geomParams,pathCntrPosVecGnd);
    else
        x1 = x2;
%         J1 = J(x1,posVec,geomParams,pathCntrPosVecGnd);
        x2 = x3;
        J2 = J3;
        x3 = x1 + (x4-x1)*0.618033988749895;
        J3 = J(x3,posVec,geomParams,pathCntrPosVecGnd);
    end
    if x4-x1<pathVarTol/2
        break
    end
end
sNext = mod((x4+x1)/2,1);
end

function val = J(sTest,posVec,geomParams,pathCntr)
az = atan2(posVec(2),posVec(1));
el = atan2(posVec(3),sqrt(posVec(1)^2+posVec(2)^2));
pathPosVec = lemOfBooth(sTest,geomParams,pathCntr);
azP = atan2(pathPosVec(2),pathPosVec(1));
elP = atan2(pathPosVec(3),sqrt(pathPosVec(1)^2+pathPosVec(2)^2));
val = (az-azP)^2+(el-elP)^2;
end
